simulink model "QAM_Simulink"  (R2021a)
settings: Solver=VariableStepAuto  StartTime=0.0  StopTime=10.0  RelTol=1e-3
libraries: commdigbbndam3 x2, commchan3 x1, commsink2 x1, commrandsrc3 x1
settings Model: Creator=DAN  LastModifiedBy=DAN

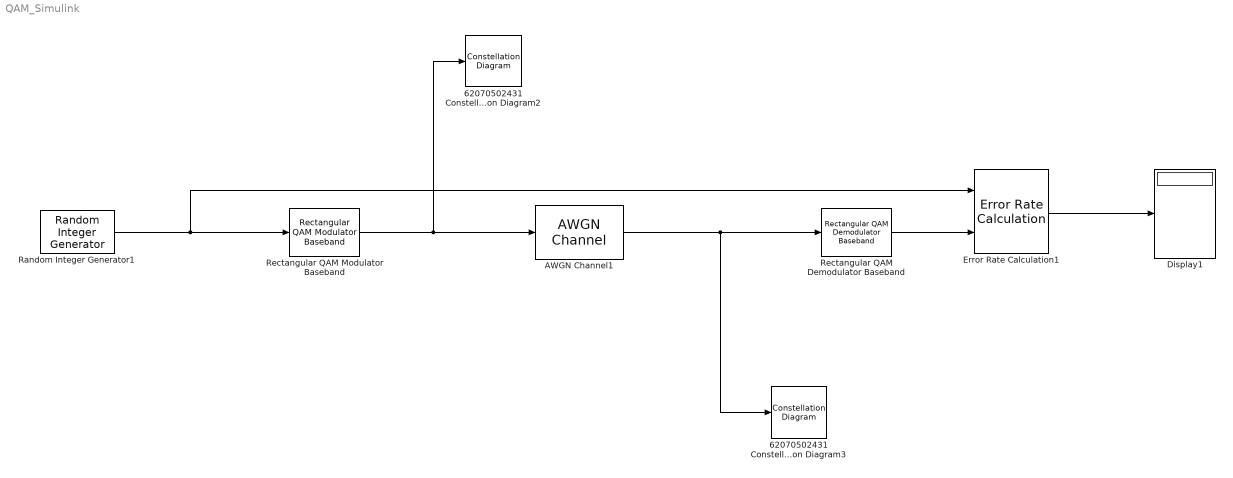
== system QAM_Simulink ==
  62070502431 Constellation Diagram2 : ConstellationDiagram
  62070502431 Constellation Diagram3 : ConstellationDiagram
  AWGN Channel1 : commchan3/AWGN Channel  InputProcessing=Columns as channels (frame based)  seed=67  noiseMode="Signal to noise ratio  (Eb/No)"  EbNodB=10  EsNodB=10  SNRdB=10  bitsPerSym=4  Ps=1  Tsym=1e-6  variance=1
  Display1 : Display
  Error Rate Calculation1 : commsink2/Error Rate Calculation  N=0  st_delay=0  cp_mode=Entire frame  subframe=[]  PMode=Port  WsName=ErrorVec  RsMode2=off  stop=off  numErr=100  maxBits=1e6
  Random Integer Generator1 : commrandsrc3/Random Integer Generator  SetSize=16  SeedSource=Auto  Seed=0  SampleTime=1e-6  SamplesPerFrame=1024  OutputDataType=double  SimulateUsing=Interpreted execution
  Rectangular QAM Demodulator Baseband : commdigbbndam3/Rectangular QAM Demodulator Baseband  M=16  OutType=Integer  DecType=Hard decision  VarSource=Dialog  Variance=1  Dec=Gray  Mapping=[0:15]  PowType=Peak Power  MinDist=2  AvgPow=1  PeakPow=1  Ph=0  outDtype1=Inherit via internal rule  outDtype2=Inherit via internal rule  derotateFactorWordLen=16  derotateFactorDataTypeStr=Inherit: Same word length as input  derotateFactorLastDataTypeStr=Inherit: Same word length as input  denormFactorWordLen=16  denormFactorDataTypeStr=Inherit: Same word length as input  denormFactorLastDataTypeStr=Inherit: Same word length as input  prodOutWordLen=32  prodOutOverflowMode=Wrap  prodOutRoundingMode=Floor  prodOutOvFlMode=off  prodOutOvFlModeLastStrValue=off  sumWordLen=32
  Rectangular QAM Modulator Baseband : commdigbbndam3/Rectangular QAM Modulator Baseband  M=16  InType=Integer  Enc=Gray  Mapping=[0:15]  PowType=Peak Power  MinDist=2  AvgPow=1  PeakPow=1  Ph=0  outDtype=double  outWordLen=16  outUDDataType=sfix(16)  outFracLenMode=Best precision  outFracLen=15  outDataTypeStr=double  outLastDataTypeStr=double
  wires:
  Rectangular QAM Demodulator Baseband/1 -> Error Rate Calculation1/2
  Rectangular QAM Modulator Baseband/1 -> 62070502431 Constellation Diagram2/1, AWGN Channel1/1
  Random Integer Generator1/1 -> Rectangular QAM Modulator Baseband/1, Error Rate Calculation1/1
  AWGN Channel1/1 -> Rectangular QAM Demodulator Baseband/1, 62070502431 Constellation Diagram3/1
  Error Rate Calculation1/1 -> Display1/1
